simulink model "MIL_VehicleTestEnvironment_MG_DCT_1"  (Simulink 10.0)
settings: Solver=ode4  StartTime=0.0  StopTime=20  FixedStep=0.001  MaxStep=0.005  RelTol=1e-3  EnableMultiTasking=on
undefined symbols (not defined in the file or in its folder): Clu1FricCoefMap, Clu2FricCoefMap, CluSoln1LineI, CluSoln1LineP, CluSoln2LineI, CluSoln2LineP, DiffDampCoef, EngFuelCnsPerSecMapCns, EngFuelCnsPerSecMapSpdIndx, EngFuelCnsPerSecMapThrtIndx, EngIdleSpd, EngSpdMax, EngTqExtChartc, EngTqMapSpdIndx, EngTqMapThrtIndx, EngTqMapTq, EngTqMax, Fork13ActrAr, Fork1PosnA, Fork1PosnB, Fork1PosnNeut, Fork1PosnSyncA, Fork1PosnSyncB, Fork24ActrAr, Fork2PosnA, Fork2PosnB, Fork2PosnNeut, Fork2PosnSyncA, Fork2PosnSyncB, Fork3PosnA, Fork3PosnB, Fork3PosnNeut, Fork3PosnSyncA, Fork3PosnSyncB, Fork4PosnA, Fork4PosnB, Fork4PosnNeut, Fork4PosnSyncA, Fork4PosnSyncB, Fork6RActrAr, ForkN5ActrAr, GearRat, HalfShafInrt, IdleGearInrt, InpShaf1DampCoef, InpShaf2DampCoef, OutpShaf1DampCoef, OutpShaf2DampCoef, ShiftSoln1LineI, ShiftSoln1LineP, ShiftSoln2LineI, ShiftSoln2LineP, SynrDiaBig, SynrDplDog, SynrDplEngd, SynrDplFinshd, SynrDplSync, SynrFricCoef, VBS1R, VBS2R ... (+6)
libraries: fl_lib x71, nesl_utility x34, sdl_lib x20, fl_ps_legacy_lib x8, simulink x5
(part 2 of 2)

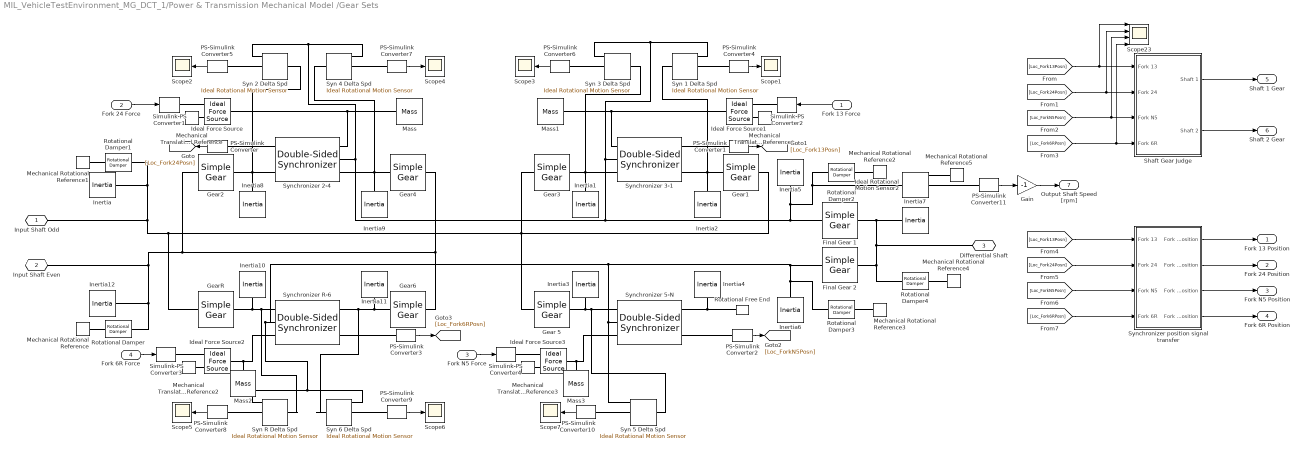
== system MIL_VehicleTestEnvironment_MG_DCT_1/Power & Transmission Mechanical Model /Gear Sets ==
  Fork 13 Force : Inport
  Fork 24 Force : Inport  Port=2
  Fork N5 Force : Inport  Port=3
  Fork 6R Force : Inport  Port=4
  Final Gear 1 : sdl_lib/Gears/Simple Gear  ratio=FinlGearRat1  rotation_direction=2  friction_model=1  T_noload=0.1 N*m  T_nom=5 N*m  efficiency_nom=0.8  efficiency=0.8  mu_visc=[ 0 0 ] N*m/(rad/s)  w_thr=0.01 rad/s  pwr_thr=0.001 W  enable_faults=simscape.enum.onoff.off  efficiency_fault=0.05  external_fault=simscape.enum.onoff.off  temporal_fault=simscape.enum.onoff.off  fault_time=5 s  fault_angles=pi / 12 rad  report_fault=1  temperature_TLU=[280, 300, 320] K  load_TLU=[1, 5, 10] N*m  efficiency_TLU=[.95, .9, .85]  efficiency_TLU2=[.85, .8, .75; .95, .9, .85; .85, .8, .7]  thermal_mass=50 J/K  T_init=300 K
  Final Gear 2 : sdl_lib/Gears/Simple Gear  ratio=FinlGearRat2  rotation_direction=2  friction_model=1  T_noload=0.1 N*m  T_nom=5 N*m  efficiency_nom=0.8  efficiency=0.8  mu_visc=[ 0 0 ] N*m/(rad/s)  w_thr=0.01 rad/s  pwr_thr=0.001 W  enable_faults=simscape.enum.onoff.off  efficiency_fault=0.05  external_fault=simscape.enum.onoff.off  temporal_fault=simscape.enum.onoff.off  fault_time=5 s  fault_angles=pi / 12 rad  report_fault=1  temperature_TLU=[280, 300, 320] K  load_TLU=[1, 5, 10] N*m  efficiency_TLU=[.95, .9, .85]  efficiency_TLU2=[.85, .8, .75; .95, .9, .85; .85, .8, .7]  thermal_mass=50 J/K  T_init=300 K
  Gain : Gain  Gain=-1
  Gear 5 : sdl_lib/Gears/Simple Gear  ratio=GearRat(5)  rotation_direction=2  friction_model=1  T_noload=0.1 N*m  T_nom=5 N*m  efficiency_nom=0.8  efficiency=0.8  mu_visc=[ 0 0 ] N*m/(rad/s)  w_thr=0.01 rad/s  pwr_thr=0.001 W  enable_faults=simscape.enum.onoff.off  efficiency_fault=0.05  external_fault=simscape.enum.onoff.off  temporal_fault=simscape.enum.onoff.off  fault_time=5 s  fault_angles=pi / 12 rad  report_fault=1  temperature_TLU=[280, 300, 320] K  load_TLU=[1, 5, 10] N*m  efficiency_TLU=[.95, .9, .85]  efficiency_TLU2=[.85, .8, .75; .95, .9, .85; .85, .8, .7]  thermal_mass=50 J/K  T_init=300 K
  Gear1 : sdl_lib/Gears/Simple Gear  ratio=GearRat(1)  rotation_direction=2  friction_model=1  T_noload=0.1 N*m  T_nom=5 N*m  efficiency_nom=0.8  efficiency=0.8  mu_visc=[ 0 0 ] N*m/(rad/s)  w_thr=0.01 rad/s  pwr_thr=0.001 W  enable_faults=simscape.enum.onoff.off  efficiency_fault=0.05  external_fault=simscape.enum.onoff.off  temporal_fault=simscape.enum.onoff.off  fault_time=5 s  fault_angles=pi / 12 rad  report_fault=1  temperature_TLU=[280, 300, 320] K  load_TLU=[1, 5, 10] N*m  efficiency_TLU=[.95, .9, .85]  efficiency_TLU2=[.85, .8, .75; .95, .9, .85; .85, .8, .7]  thermal_mass=50 J/K  T_init=300 K
  Gear2 : sdl_lib/Gears/Simple Gear  ratio=GearRat(2)  rotation_direction=2  friction_model=1  T_noload=0.1 N*m  T_nom=5 N*m  efficiency_nom=0.8  efficiency=0.8  mu_visc=[ 0 0 ] N*m/(rad/s)  w_thr=0.01 rad/s  pwr_thr=0.001 W  enable_faults=simscape.enum.onoff.off  efficiency_fault=0.05  external_fault=simscape.enum.onoff.off  temporal_fault=simscape.enum.onoff.off  fault_time=5 s  fault_angles=pi / 12 rad  report_fault=1  temperature_TLU=[280, 300, 320] K  load_TLU=[1, 5, 10] N*m  efficiency_TLU=[.95, .9, .85]  efficiency_TLU2=[.85, .8, .75; .95, .9, .85; .85, .8, .7]  thermal_mass=50 J/K  T_init=300 K
  Gear3 : sdl_lib/Gears/Simple Gear  ratio=GearRat(3)  rotation_direction=2  friction_model=1  T_noload=0.1 N*m  T_nom=5 N*m  efficiency_nom=0.8  efficiency=0.8  mu_visc=[ 0 0 ] N*m/(rad/s)  w_thr=0.01 rad/s  pwr_thr=0.001 W  enable_faults=simscape.enum.onoff.off  efficiency_fault=0.05  external_fault=simscape.enum.onoff.off  temporal_fault=simscape.enum.onoff.off  fault_time=5 s  fault_angles=pi / 12 rad  report_fault=1  temperature_TLU=[280, 300, 320] K  load_TLU=[1, 5, 10] N*m  efficiency_TLU=[.95, .9, .85]  efficiency_TLU2=[.85, .8, .75; .95, .9, .85; .85, .8, .7]  thermal_mass=50 J/K  T_init=300 K
  Gear4 : sdl_lib/Gears/Simple Gear  ratio=GearRat(4)  rotation_direction=2  friction_model=1  T_noload=0.1 N*m  T_nom=5 N*m  efficiency_nom=0.8  efficiency=0.8  mu_visc=[ 0 0 ] N*m/(rad/s)  w_thr=0.01 rad/s  pwr_thr=0.001 W  enable_faults=simscape.enum.onoff.off  efficiency_fault=0.05  external_fault=simscape.enum.onoff.off  temporal_fault=simscape.enum.onoff.off  fault_time=5 s  fault_angles=pi / 12 rad  report_fault=1  temperature_TLU=[280, 300, 320] K  load_TLU=[1, 5, 10] N*m  efficiency_TLU=[.95, .9, .85]  efficiency_TLU2=[.85, .8, .75; .95, .9, .85; .85, .8, .7]  thermal_mass=50 J/K  T_init=300 K
  Gear6 : sdl_lib/Gears/Simple Gear  ratio=GearRat(6)  rotation_direction=2  friction_model=1  T_noload=0.1 N*m  T_nom=5 N*m  efficiency_nom=0.8  efficiency=0.8  mu_visc=[ 0 0 ] N*m/(rad/s)  w_thr=0.01 rad/s  pwr_thr=0.001 W  enable_faults=simscape.enum.onoff.off  efficiency_fault=0.05  external_fault=simscape.enum.onoff.off  temporal_fault=simscape.enum.onoff.off  fault_time=5 s  fault_angles=pi / 12 rad  report_fault=1  temperature_TLU=[280, 300, 320] K  load_TLU=[1, 5, 10] N*m  efficiency_TLU=[.95, .9, .85]  efficiency_TLU2=[.85, .8, .75; .95, .9, .85; .85, .8, .7]  thermal_mass=50 J/K  T_init=300 K
  GearR : sdl_lib/Gears/Simple Gear  ratio=GearRat(7)  rotation_direction=1  friction_model=1  T_noload=0.1 N*m  T_nom=5 N*m  efficiency_nom=0.8  efficiency=0.8  mu_visc=[ 0 0 ] N*m/(rad/s)  w_thr=0.01 rad/s  pwr_thr=0.001 W  enable_faults=simscape.enum.onoff.off  efficiency_fault=0.05  external_fault=simscape.enum.onoff.off  temporal_fault=simscape.enum.onoff.off  fault_time=5 s  fault_angles=pi / 12 rad  report_fault=1  temperature_TLU=[280, 300, 320] K  load_TLU=[1, 5, 10] N*m  efficiency_TLU=[.95, .9, .85]  efficiency_TLU2=[.85, .8, .75; .95, .9, .85; .85, .8, .7]  thermal_mass=50 J/K  T_init=300 K
  Ideal Force Source{,1..3} (4 alike) : fl_lib/Mechanical/Mechanical Sources/Ideal Force Source
  Ideal Rotational Motion Sensor2 : fl_lib/Mechanical/Mechanical Sensors/Ideal Rotational Motion Sensor  wrap_angle=simscape.enum.onoff.off  offset=0 rad
  Inertia : fl_lib/Mechanical/Rotational Elements/Inertia  inertia=InpShaf1Inrt kg*m^2  w_specify=off  w_priority=High  w=0 rad/s  w_nominal_specify=off  w_nominal_unit=rad/s  w_nominal_value=1  t_specify=off  t_priority=High  t=0 N*m  t_nominal_specify=off  t_nominal_unit=N*m  t_nominal_value=1
  Inertia1 : fl_lib/Mechanical/Rotational Elements/Inertia  inertia=IdleGearInrt(3) kg*m^2  w_specify=off  w_priority=High  w=0 rad/s  w_nominal_specify=off  w_nominal_unit=rad/s  w_nominal_value=1  t_specify=off  t_priority=High  t=0 N*m  t_nominal_specify=off  t_nominal_unit=N*m  t_nominal_value=1
  Inertia10 : fl_lib/Mechanical/Rotational Elements/Inertia  inertia=IdleGearInrt(7) kg*m^2  w_specify=off  w_priority=High  w=0 rad/s  w_nominal_specify=off  w_nominal_unit=rad/s  w_nominal_value=1  t_specify=off  t_priority=High  t=0 N*m  t_nominal_specify=off  t_nominal_unit=N*m  t_nominal_value=1
  Inertia11 : fl_lib/Mechanical/Rotational Elements/Inertia  inertia=IdleGearInrt(6) kg*m^2  w_specify=off  w_priority=High  w=0 rad/s  w_nominal_specify=off  w_nominal_unit=rad/s  w_nominal_value=1  t_specify=off  t_priority=High  t=0 N*m  t_nominal_specify=off  t_nominal_unit=N*m  t_nominal_value=1
  Inertia12 : fl_lib/Mechanical/Rotational Elements/Inertia  inertia=InpShaf2Inrt kg*m^2  w_specify=off  w_priority=High  w=0 rad/s  w_nominal_specify=off  w_nominal_unit=rad/s  w_nominal_value=1  t_specify=off  t_priority=High  t=0 N*m  t_nominal_specify=off  t_nominal_unit=N*m  t_nominal_value=1
  Inertia2 : fl_lib/Mechanical/Rotational Elements/Inertia  inertia=IdleGearInrt(1) kg*m^2  w_specify=off  w_priority=High  w=0 rad/s  w_nominal_specify=off  w_nominal_unit=rad/s  w_nominal_value=1  t_specify=off  t_priority=High  t=0 N*m  t_nominal_specify=off  t_nominal_unit=N*m  t_nominal_value=1
  Inertia3 : fl_lib/Mechanical/Rotational Elements/Inertia  inertia=IdleGearInrt(5) kg*m^2  w_specify=off  w_priority=High  w=0 rad/s  w_nominal_specify=off  w_nominal_unit=rad/s  w_nominal_value=1  t_specify=off  t_priority=High  t=0 N*m  t_nominal_specify=off  t_nominal_unit=N*m  t_nominal_value=1
  Inertia4 : fl_lib/Mechanical/Rotational Elements/Inertia  inertia=0.001 kg*m^2  w_specify=off  w_priority=High  w=0 rad/s  w_nominal_specify=off  w_nominal_unit=rad/s  w_nominal_value=1  t_specify=off  t_priority=High  t=0 N*m  t_nominal_specify=off  t_nominal_unit=N*m  t_nominal_value=1
  Inertia5 : fl_lib/Mechanical/Rotational Elements/Inertia  inertia=OutpShaf1Inrt kg*m^2  w_specify=off  w_priority=High  w=0 rad/s  w_nominal_specify=off  w_nominal_unit=rad/s  w_nominal_value=1  t_specify=off  t_priority=High  t=0 N*m  t_nominal_specify=off  t_nominal_unit=N*m  t_nominal_value=1
  Inertia6 : fl_lib/Mechanical/Rotational Elements/Inertia  inertia=OutpShaf2Inrt kg*m^2  w_specify=off  w_priority=High  w=0 rad/s  w_nominal_specify=off  w_nominal_unit=rad/s  w_nominal_value=1  t_specify=off  t_priority=High  t=0 N*m  t_nominal_specify=off  t_nominal_unit=N*m  t_nominal_value=1
  Inertia7 : fl_lib/Mechanical/Rotational Elements/Inertia  inertia=DiffInrt kg*m^2  w_specify=off  w_priority=High  w=0 rad/s  w_nominal_specify=off  w_nominal_unit=rad/s  w_nominal_value=1  t_specify=off  t_priority=High  t=0 N*m  t_nominal_specify=off  t_nominal_unit=N*m  t_nominal_value=1
  Inertia8 : fl_lib/Mechanical/Rotational Elements/Inertia  inertia=IdleGearInrt(2) kg*m^2  w_specify=off  w_priority=High  w=0 rad/s  w_nominal_specify=off  w_nominal_unit=rad/s  w_nominal_value=1  t_specify=off  t_priority=High  t=0 N*m  t_nominal_specify=off  t_nominal_unit=N*m  t_nominal_value=1
  Inertia9 : fl_lib/Mechanical/Rotational Elements/Inertia  inertia=IdleGearInrt(4) kg*m^2  w_specify=off  w_priority=High  w=0 rad/s  w_nominal_specify=off  w_nominal_unit=rad/s  w_nominal_value=1  t_specify=off  t_priority=High  t=0 N*m  t_nominal_specify=off  t_nominal_unit=N*m  t_nominal_value=1
  Mass{,1..3} (4 alike) : fl_lib/Mechanical/Translational Elements/Mass  mass=1 kg  v_specify=off  v_priority=High  v=0 m/s  v_nominal_specify=off  v_nominal_unit=m/s  v_nominal_value=1  f_specify=off  f_priority=High  f=0 N  f_nominal_specify=off  f_nominal_unit=N  f_nominal_value=1
  Mechanical Rotational Reference{,1..5} (6 alike) : fl_lib/Mechanical/Rotational Elements/Mechanical Rotational Reference
  Mechanical Translational Reference{,1..3} (4 alike) : fl_lib/Mechanical/Translational Elements/Mechanical Translational Reference
  PS-Simulink Converter{,1..3} (4 alike) : nesl_utility/PS-Simulink Converter  PhysicalDomain=network_engine_domain  SubClassName=ps_output  LeftPortType=input  RightPortType=output  PseudoPeriodic=off  Frequencies=[]  Unit=mm  AffineConversion=off
  PS-Simulink Converter{4..11} (8 alike) : nesl_utility/PS-Simulink Converter  PhysicalDomain=network_engine_domain  SubClassName=ps_output  LeftPortType=input  RightPortType=output  PseudoPeriodic=off  Frequencies=[]  Unit=rpm  AffineConversion=off
  Rotational Damper : fl_lib/Mechanical/Rotational Elements/Rotational Damper  D=InpShaf2DampCoef N*m/(rad/s)  w_specify=off  w_priority=High  w=0 rad/s  w_nominal_specify=off  w_nominal_unit=rad/s  w_nominal_value=1  t_specify=off  t_priority=High  t=0 N*m  t_nominal_specify=off  t_nominal_unit=N*m  t_nominal_value=1
  Rotational Damper1 : fl_lib/Mechanical/Rotational Elements/Rotational Damper  D=InpShaf1DampCoef N*m/(rad/s)  w_specify=off  w_priority=High  w=0 rad/s  w_nominal_specify=off  w_nominal_unit=rad/s  w_nominal_value=1  t_specify=off  t_priority=High  t=0 N*m  t_nominal_specify=off  t_nominal_unit=N*m  t_nominal_value=1
  Rotational Damper2 : fl_lib/Mechanical/Rotational Elements/Rotational Damper  D=OutpShaf1DampCoef N*m/(rad/s)  w_specify=off  w_priority=High  w=0 rad/s  w_nominal_specify=off  w_nominal_unit=rad/s  w_nominal_value=1  t_specify=off  t_priority=High  t=0 N*m  t_nominal_specify=off  t_nominal_unit=N*m  t_nominal_value=1
  Rotational Damper3 : fl_lib/Mechanical/Rotational Elements/Rotational Damper  D=OutpShaf2DampCoef N*m/(rad/s)  w_specify=off  w_priority=High  w=0 rad/s  w_nominal_specify=off  w_nominal_unit=rad/s  w_nominal_value=1  t_specify=off  t_priority=High  t=0 N*m  t_nominal_specify=off  t_nominal_unit=N*m  t_nominal_value=1
  Rotational Damper4 : fl_lib/Mechanical/Rotational Elements/Rotational Damper  D=DiffDampCoef N*m/(rad/s)  w_specify=off  w_priority=High  w=0 rad/s  w_nominal_specify=off  w_nominal_unit=rad/s  w_nominal_value=1  t_specify=off  t_priority=High  t=0 N*m  t_nominal_specify=off  t_nominal_unit=N*m  t_nominal_value=1
  Rotational Free End : fl_lib/Mechanical/Rotational Elements/Rotational Free End  w_specify=off  w_priority=None  w=0 rad/s  w_nominal_specify=off  w_nominal_unit=rad/s  w_nominal_value=1
      settings: SourceProductBaseCode=SS
  Scope{1..7} (7 alike) : Scope
  Scope23 : Scope  NumInputPorts=4
  "Shaft Gear Judge " : Subsystem
  Simulink-PS Converter{1..4} (4 alike) : nesl_utility/Simulink-PS Converter  PhysicalDomain=network_engine_domain  SubClassName=ps_input  LeftPortType=input  RightPortType=output  PseudoPeriodic=off  Frequencies=[]  NoiseDistribution=none  NoiseParameters=[]  Unit=N  AffineConversion=off  FilteringAndDerivatives=zero  SimscapeFilterOrder=1  InputFilterTimeConstant=0.001  UdotUserProvided=1
  Syn 1 Delta Spd : fl_lib/Mechanical/Mechanical Sensors/Ideal Rotational Motion Sensor  wrap_angle=simscape.enum.onoff.off  offset=0 rad
  Syn 2 Delta Spd : fl_lib/Mechanical/Mechanical Sensors/Ideal Rotational Motion Sensor  wrap_angle=simscape.enum.onoff.off  offset=0 rad
  Syn 3 Delta Spd : fl_lib/Mechanical/Mechanical Sensors/Ideal Rotational Motion Sensor  wrap_angle=simscape.enum.onoff.off  offset=0 rad
  Syn 4 Delta Spd : fl_lib/Mechanical/Mechanical Sensors/Ideal Rotational Motion Sensor  wrap_angle=simscape.enum.onoff.off  offset=0 rad
  Syn 5 Delta Spd : fl_lib/Mechanical/Mechanical Sensors/Ideal Rotational Motion Sensor  wrap_angle=simscape.enum.onoff.off  offset=0 rad
  Syn 6 Delta Spd : fl_lib/Mechanical/Mechanical Sensors/Ideal Rotational Motion Sensor  wrap_angle=simscape.enum.onoff.off  offset=0 rad
  Syn R Delta Spd : fl_lib/Mechanical/Mechanical Sensors/Ideal Rotational Motion Sensor  wrap_angle=simscape.enum.onoff.off  offset=0 rad
  Synchronizer 2-4 : sdl_lib/Clutches/Double-Sided Synchronizer  d_o=SynrDiaBig*2 m  d_i=SynrDiaSmal m  theta=SynrConeAngl deg  friction_model=2  mu_w_vector=SynrFricCoef(:,1) rad/s  mu_temperature_TLU=[280, 300, 320] K  mu_static=SynrFricCoef(1,2)+0.05  mu_static_vector=[.4, .38, .36]  mu_coulomb=0.3  mu_coulomb_vector=SynrFricCoef(:,2)  mu_coulomb_temp_vector=[.3, .28, .25]  mu_coulomb_matrix=[.34, .32, .3; .3, .28, .25; .25, .2, .15]  mu_interp_method=1  mu_extrap_method=1  w_tol=0.001 rad/s  force_min=1 N  model=1  max_torque=1000 N*m  torque_temperature_TLU=[280, 300, 320] K  max_torque_vector=[1000, 1050, 1000] N*m  torque_interp_method=1  torque_extrap_method=1  radius=200 mm  n_teeth=6  clutch_backlash=10 deg  clutch_stiffness=1e+7 N*m/rad  clutch_damping=100 N*m/(rad/s)  fric_coeff=0.05  peak_force=SynrDetnForMax N  width=SynrNotchWidth mm  detent_visc_fric_transl=0.1 N/(m/s)  friction_ratio=0.01  v_thr=0.05 m/s  engagement_speed=1 rpm  dog_clutch_ring_hub_gap=SynrDplDog mm  engagement_overlap=SynrDplEngd-SynrDplDog mm  tooth_height=SynrDplFinshd-SynrDplDog mm  cone_clutch_ring_hub_gap=SynrDplSync mm  dog_clutch_transl_stiffness=1e+6 N/m  cone_clutch_transl_stiffness=1e+6 N/m  dog_clutch_transl_damping=1000 N/(m/s)  cone_clutch_transl_damping=1000 N/(m/s)  dog_clutch_visc_fric_transl=SynrVcosFricCoeff N/(m/s)  initial_state_locked=3  dog_clutch_init_pos=0 mm  cone_clutch_init_pos=0 mm  init_rel_angle_A=0 deg  init_rel_angle_B=0 deg  thermal_mass=100 kJ/K  T_init=300 K
      settings: SourceProductBaseCode=LD  InternalSimscapePortConfiguration="{\"Bottom\":[],\"Left\":[{\"id\":\"S\",\"label\":\"S\",\"type\":\"foundation.mechanical.translational.translational\"},{\"id\":\"R\",\"label\":\"R\",\"type\":\"foundation.mechanical.rotational.rotational\"},{\"id\":\"HA\",\"label\":\"HA\",\"type\":\"foundation.mechanical.rotational.rotational\"}],\"Right\":[{\"id\":\"X1\",\"label\":\"X1\",\"type\":\"output\"},{\"id\":\"X2\",\"label\":\"X2\",\"type\":\"output\"},{\"id\":\"HB\",\"label\":\"HB\",\"type\":\"foundation.mechanical.rotational.rotational\"}],\"Top\":[]}"
  Synchronizer 3-1 : sdl_lib/Clutches/Double-Sided Synchronizer  d_o=SynrDiaBig m  d_i=SynrDiaSmal m  theta=SynrConeAngl deg  friction_model=2  mu_w_vector=SynrFricCoef(:,1) rad/s  mu_temperature_TLU=[280, 300, 320] K  mu_static=SynrFricCoef(1,2)+0.05  mu_static_vector=[.4, .38, .36]  mu_coulomb=0.3  mu_coulomb_vector=SynrFricCoef(:,2)  mu_coulomb_temp_vector=[.3, .28, .25]  mu_coulomb_matrix=[.34, .32, .3; .3, .28, .25; .25, .2, .15]  mu_interp_method=1  mu_extrap_method=1  w_tol=0.001 rad/s  force_min=1 N  model=1  max_torque=1000 N*m  torque_temperature_TLU=[280, 300, 320] K  max_torque_vector=[1000, 1050, 1000] N*m  torque_interp_method=1  torque_extrap_method=1  radius=200 mm  n_teeth=6  clutch_backlash=10 deg  clutch_stiffness=1e+7 N*m/rad  clutch_damping=100 N*m/(rad/s)  fric_coeff=0.05  peak_force=SynrDetnForMax N  width=SynrNotchWidth mm  detent_visc_fric_transl=0.1 N/(m/s)  friction_ratio=0.01  v_thr=0.05 m/s  engagement_speed=1 rpm  dog_clutch_ring_hub_gap=SynrDplDog mm  engagement_overlap=SynrDplEngd-SynrDplDog mm  tooth_height=SynrDplFinshd-SynrDplDog mm  cone_clutch_ring_hub_gap=SynrDplSync mm  dog_clutch_transl_stiffness=1e+6 N/m  cone_clutch_transl_stiffness=1e+6 N/m  dog_clutch_transl_damping=1000 N/(m/s)  cone_clutch_transl_damping=1000 N/(m/s)  dog_clutch_visc_fric_transl=SynrVcosFricCoeff N/(m/s)  initial_state_locked=3  dog_clutch_init_pos=0 mm  cone_clutch_init_pos=0 mm  init_rel_angle_A=0 deg  init_rel_angle_B=0 deg  thermal_mass=100 kJ/K  T_init=300 K
      settings: SourceProductBaseCode=LD  InternalSimscapePortConfiguration="{\"Bottom\":[],\"Left\":[{\"id\":\"S\",\"label\":\"S\",\"type\":\"foundation.mechanical.translational.translational\"},{\"id\":\"R\",\"label\":\"R\",\"type\":\"foundation.mechanical.rotational.rotational\"},{\"id\":\"HA\",\"label\":\"HA\",\"type\":\"foundation.mechanical.rotational.rotational\"}],\"Right\":[{\"id\":\"X1\",\"label\":\"X1\",\"type\":\"output\"},{\"id\":\"X2\",\"label\":\"X2\",\"type\":\"output\"},{\"id\":\"HB\",\"label\":\"HB\",\"type\":\"foundation.mechanical.rotational.rotational\"}],\"Top\":[]}"
  Synchronizer 5-N : sdl_lib/Clutches/Double-Sided Synchronizer  d_o=SynrDiaBig m  d_i=SynrDiaSmal m  theta=SynrConeAngl deg  friction_model=2  mu_w_vector=SynrFricCoef(:,1) rad/s  mu_temperature_TLU=[280, 300, 320] K  mu_static=SynrFricCoef(1,2)+0.05  mu_static_vector=[.4, .38, .36]  mu_coulomb=0.3  mu_coulomb_vector=SynrFricCoef(:,2)  mu_coulomb_temp_vector=[.3, .28, .25]  mu_coulomb_matrix=[.34, .32, .3; .3, .28, .25; .25, .2, .15]  mu_interp_method=1  mu_extrap_method=1  w_tol=0.001 rad/s  force_min=1 N  model=1  max_torque=1000 N*m  torque_temperature_TLU=[280, 300, 320] K  max_torque_vector=[1000, 1050, 1000] N*m  torque_interp_method=1  torque_extrap_method=1  radius=200 mm  n_teeth=6  clutch_backlash=10 deg  clutch_stiffness=1e+7 N*m/rad  clutch_damping=100 N*m/(rad/s)  fric_coeff=0.05  peak_force=SynrDetnForMax N  width=SynrNotchWidth mm  detent_visc_fric_transl=0.1 N/(m/s)  friction_ratio=0.01  v_thr=0.05 m/s  engagement_speed=1 rpm  dog_clutch_ring_hub_gap=SynrDplDog mm  engagement_overlap=SynrDplEngd-SynrDplDog mm  tooth_height=SynrDplFinshd-SynrDplDog mm  cone_clutch_ring_hub_gap=SynrDplSync mm  dog_clutch_transl_stiffness=1e+6 N/m  cone_clutch_transl_stiffness=1e+6 N/m  dog_clutch_transl_damping=1000 N/(m/s)  cone_clutch_transl_damping=1000 N/(m/s)  dog_clutch_visc_fric_transl=SynrVcosFricCoeff N/(m/s)  initial_state_locked=3  dog_clutch_init_pos=0 mm  cone_clutch_init_pos=0 mm  init_rel_angle_A=0 deg  init_rel_angle_B=0 deg  thermal_mass=100 kJ/K  T_init=300 K
      settings: SourceProductBaseCode=LD  InternalSimscapePortConfiguration="{\"Bottom\":[],\"Left\":[{\"id\":\"S\",\"label\":\"S\",\"type\":\"foundation.mechanical.translational.translational\"},{\"id\":\"R\",\"label\":\"R\",\"type\":\"foundation.mechanical.rotational.rotational\"},{\"id\":\"HA\",\"label\":\"HA\",\"type\":\"foundation.mechanical.rotational.rotational\"}],\"Right\":[{\"id\":\"X1\",\"label\":\"X1\",\"type\":\"output\"},{\"id\":\"X2\",\"label\":\"X2\",\"type\":\"output\"},{\"id\":\"HB\",\"label\":\"HB\",\"type\":\"foundation.mechanical.rotational.rotational\"}],\"Top\":[]}"
  Synchronizer R-6 : sdl_lib/Clutches/Double-Sided Synchronizer  d_o=SynrDiaBig m  d_i=SynrDiaSmal m  theta=SynrConeAngl deg  friction_model=2  mu_w_vector=SynrFricCoef(:,1) rad/s  mu_temperature_TLU=[280, 300, 320] K  mu_static=SynrFricCoef(1,2)+0.05  mu_static_vector=[.4, .38, .36]  mu_coulomb=0.3  mu_coulomb_vector=SynrFricCoef(:,2)  mu_coulomb_temp_vector=[.3, .28, .25]  mu_coulomb_matrix=[.34, .32, .3; .3, .28, .25; .25, .2, .15]  mu_interp_method=1  mu_extrap_method=1  w_tol=0.001 rad/s  force_min=1 N  model=1  max_torque=1000 N*m  torque_temperature_TLU=[280, 300, 320] K  max_torque_vector=[1000, 1050, 1000] N*m  torque_interp_method=1  torque_extrap_method=1  radius=200 mm  n_teeth=6  clutch_backlash=10 deg  clutch_stiffness=1e+7 N*m/rad  clutch_damping=100 N*m/(rad/s)  fric_coeff=0.05  peak_force=SynrDetnForMax N  width=SynrNotchWidth mm  detent_visc_fric_transl=0.1 N/(m/s)  friction_ratio=0.01  v_thr=0.05 m/s  engagement_speed=1 rpm  dog_clutch_ring_hub_gap=SynrDplDog mm  engagement_overlap=SynrDplEngd-SynrDplDog mm  tooth_height=SynrDplFinshd-SynrDplDog mm  cone_clutch_ring_hub_gap=SynrDplSync mm  dog_clutch_transl_stiffness=1e+6 N/m  cone_clutch_transl_stiffness=1e+6 N/m  dog_clutch_transl_damping=1000 N/(m/s)  cone_clutch_transl_damping=1000 N/(m/s)  dog_clutch_visc_fric_transl=SynrVcosFricCoeff N/(m/s)  initial_state_locked=3  dog_clutch_init_pos=0 mm  cone_clutch_init_pos=0 mm  init_rel_angle_A=0 deg  init_rel_angle_B=0 deg  thermal_mass=100 kJ/K  T_init=300 K
      settings: SourceProductBaseCode=LD  InternalSimscapePortConfiguration="{\"Bottom\":[],\"Left\":[{\"id\":\"S\",\"label\":\"S\",\"type\":\"foundation.mechanical.translational.translational\"},{\"id\":\"R\",\"label\":\"R\",\"type\":\"foundation.mechanical.rotational.rotational\"},{\"id\":\"HA\",\"label\":\"HA\",\"type\":\"foundation.mechanical.rotational.rotational\"}],\"Right\":[{\"id\":\"X1\",\"label\":\"X1\",\"type\":\"output\"},{\"id\":\"X2\",\"label\":\"X2\",\"type\":\"output\"},{\"id\":\"HB\",\"label\":\"HB\",\"type\":\"foundation.mechanical.rotational.rotational\"}],\"Top\":[]}"
  Synchronizer position signal transfer : Subsystem
  Input Shaft Odd : PMIOPort  Side=Left
  Input Shaft Even : PMIOPort  Port=2  Side=Left
  Differential Shaft : PMIOPort  Port=3  Side=Right
  Fork 13 Position : Outport  VectorParamsAs1DForOutWhenUnconnected=off
  Fork 24 Position : Outport  Port=2  VectorParamsAs1DForOutWhenUnconnected=off
  Fork N5 Position : Outport  Port=3  VectorParamsAs1DForOutWhenUnconnected=off
  Fork 6R Position : Outport  Port=4  VectorParamsAs1DForOutWhenUnconnected=off
  Shaft 1 Gear : Outport  Port=5  VectorParamsAs1DForOutWhenUnconnected=off
  Shaft 2 Gear : Outport  Port=6  VectorParamsAs1DForOutWhenUnconnected=off
  Output Shaft Speed [rpm] : Outport  Port=7  VectorParamsAs1DForOutWhenUnconnected=off
  wires:
  PS-Simulink Converter/1 -> [Loc_Fork24Posn]
  PS-Simulink Converter1/1 -> [Loc_Fork13Posn]
  PS-Simulink Converter2/1 -> [Loc_ForkN5Posn]
  [Loc_Fork13Posn] -> Scope23/1, "Shaft Gear Judge "/1(Fork 13)
  [Loc_Fork24Posn] -> Scope23/2, "Shaft Gear Judge "/2(Fork 24)
  [Loc_ForkN5Posn] -> Scope23/3, "Shaft Gear Judge "/3(Fork N5)
  [Loc_Fork6RPosn] -> Scope23/4, "Shaft Gear Judge "/4(Fork 6R)
  "Shaft Gear Judge "/1(Shaft 1) -> Shaft 1 Gear/1
  "Shaft Gear Judge "/2(Shaft 2) -> Shaft 2 Gear/1
  PS-Simulink Converter3/1 -> [Loc_Fork6RPosn]
  Fork 6R Force/1 -> Simulink-PS Converter3/1
  Fork N5 Force/1 -> Simulink-PS Converter4/1
  [Loc_Fork24Posn] -> Synchronizer position signal transfer/2(Fork 24)
  [Loc_ForkN5Posn] -> Synchronizer position signal transfer/3(Fork N5)
  [Loc_Fork6RPosn] -> Synchronizer position signal transfer/4(Fork 6R)
  [Loc_Fork13Posn] -> Synchronizer position signal transfer/1(Fork 13)
  Synchronizer position signal transfer/1(Fork 13 Position) -> Fork 13 Position/1
  Synchronizer position signal transfer/3(Fork N5 Position) -> Fork N5 Position/1
  Synchronizer position signal transfer/2(Fork 24 Position) -> Fork 24 Position/1
  Synchronizer position signal transfer/4(Fork 6R Position) -> Fork 6R Position/1
  PS-Simulink Converter4/1 -> Scope1/1
  PS-Simulink Converter6/1 -> Scope3/1
  PS-Simulink Converter5/1 -> Scope2/1
  PS-Simulink Converter7/1 -> Scope4/1
  PS-Simulink Converter8/1 -> Scope5/1
  PS-Simulink Converter9/1 -> Scope6/1
  PS-Simulink Converter10/1 -> Scope7/1
  Fork 24 Force/1 -> Simulink-PS Converter1/1
  Fork 13 Force/1 -> Simulink-PS Converter2/1
  PS-Simulink Converter11/1 -> Gain/1
  Gain/1 -> Output Shaft Speed [rpm]/1
  connections:
  Gear 5/LConn1 -- Gear1/LConn1 -- Gear3/LConn1 -- GearR/LConn1 -- Rotational Damper1/LConn1 -- Inertia/LConn1 -- Input Shaft Odd/RConn1
  Gear3/RConn1 -- Syn 3 Delta Spd/LConn1 -- Inertia1/LConn1 -- Synchronizer 3-1/LConn3
  Gear1/RConn1 -- Syn 1 Delta Spd/LConn1 -- Synchronizer 3-1/RConn3 -- Inertia2/LConn1
  Gear 5/RConn1 -- Syn 5 Delta Spd/LConn1 -- Synchronizer 5-N/LConn3 -- Inertia3/LConn1
  Final Gear 1/LConn1 -- Syn 2 Delta Spd/RConn1 -- Syn 4 Delta Spd/RConn1 -- Synchronizer 2-4/LConn2 -- Syn 3 Delta Spd/RConn1 -- Syn 1 Delta Spd/RConn1 -- Synchronizer 3-1/LConn2 -- Ideal Rotational Motion Sensor2/LConn1 -- Rotational Damper2/LConn1 -- Inertia5/LConn1
  Syn 6 Delta Spd/RConn1 -- Syn R Delta Spd/RConn1 -- Synchronizer R-6/LConn2 -- Syn 5 Delta Spd/RConn1 -- Synchronizer 5-N/LConn2 -- Rotational Damper3/LConn1 -- Inertia6/LConn1 -- Final Gear 2/LConn1
  Differential Shaft/RConn1 -- Final Gear 1/RConn1 -- Inertia7/LConn1 -- Rotational Damper4/LConn1 -- Final Gear 2/RConn1
  Gear4/RConn1 -- Syn 4 Delta Spd/LConn1 -- Synchronizer 2-4/LConn3 -- Inertia9/LConn1
  Synchronizer 2-4/RConn3 -- Syn 2 Delta Spd/LConn1 -- Inertia8/LConn1 -- Gear2/RConn1
  GearR/RConn1 -- Syn R Delta Spd/LConn1 -- Synchronizer R-6/LConn3 -- Inertia10/LConn1
  Syn 6 Delta Spd/LConn1 -- Synchronizer R-6/RConn3 -- Gear6/RConn1 -- Inertia11/LConn1
  Gear4/LConn1 -- Rotational Damper/LConn1 -- Inertia12/LConn1 -- Input Shaft Even/RConn1 -- Gear2/LConn1 -- Gear6/LConn1
  PS-Simulink Converter1/LConn1 -- Synchronizer 3-1/RConn1
  Synchronizer 5-N/RConn1 -- PS-Simulink Converter2/LConn1
  PS-Simulink Converter/LConn1 -- Synchronizer 2-4/RConn1
  PS-Simulink Converter3/LConn1 -- Synchronizer R-6/RConn1
  Ideal Force Source/LConn1 -- Mass/LConn1 -- Synchronizer 2-4/LConn1
  Simulink-PS Converter1/RConn1 -- Ideal Force Source/RConn1
  Mechanical Translational Reference/LConn1 -- Ideal Force Source/RConn2
  Simulink-PS Converter2/RConn1 -- Ideal Force Source1/RConn1
  Mechanical Translational Reference1/LConn1 -- Ideal Force Source1/RConn2
  Ideal Force Source1/LConn1 -- Mass1/LConn1 -- Synchronizer 3-1/LConn1
  Ideal Force Source2/LConn1 -- Mass2/LConn1 -- Synchronizer R-6/LConn1
  Simulink-PS Converter3/RConn1 -- Ideal Force Source2/RConn1
  Mechanical Translational Reference2/LConn1 -- Ideal Force Source2/RConn2
  Ideal Force Source3/LConn1 -- Synchronizer 5-N/LConn1 -- Mass3/LConn1
  Simulink-PS Converter4/RConn1 -- Ideal Force Source3/RConn1
  Mechanical Translational Reference3/LConn1 -- Ideal Force Source3/RConn2
  Rotational Free End/LConn1 -- Synchronizer 5-N/RConn3 -- Inertia4/LConn1
  Syn 1 Delta Spd/RConn2 -- PS-Simulink Converter4/LConn1
  Syn 3 Delta Spd/RConn2 -- PS-Simulink Converter6/LConn1
  Syn 2 Delta Spd/RConn2 -- PS-Simulink Converter5/LConn1
  Syn 4 Delta Spd/RConn2 -- PS-Simulink Converter7/LConn1
  Syn 6 Delta Spd/RConn2 -- PS-Simulink Converter9/LConn1
  Syn R Delta Spd/RConn2 -- PS-Simulink Converter8/LConn1
  Syn 5 Delta Spd/RConn2 -- PS-Simulink Converter10/LConn1
  Mechanical Rotational Reference/LConn1 -- Rotational Damper/RConn1
  Mechanical Rotational Reference1/LConn1 -- Rotational Damper1/RConn1
  Mechanical Rotational Reference2/LConn1 -- Rotational Damper2/RConn1
  Mechanical Rotational Reference3/LConn1 -- Rotational Damper3/RConn1
  Mechanical Rotational Reference4/LConn1 -- Rotational Damper4/RConn1
  Ideal Rotational Motion Sensor2/RConn1 -- Mechanical Rotational Reference5/LConn1
  Ideal Rotational Motion Sensor2/RConn2 -- PS-Simulink Converter11/LConn1

== system MIL_VehicleTestEnvironment_MG_DCT_1/Shift Control System/Solenoid control ==
  target current : Inport
  Constant : Constant  Value=13/VBS1R*1000
  MinMax : MinMax  Inputs=2
  actual current : Outport  VectorParamsAs1DForOutWhenUnconnected=off
  wires:
  Constant/1 -> MinMax/2
  target current/1 -> MinMax/1
  MinMax/1 -> actual current/1

== system MIL_VehicleTestEnvironment_MG_DCT_1/Shift Control System/Solenoid control1 ==
  target current : Inport
  Constant : Constant  Value=13/VBS2R*1000
  MinMax : MinMax  Inputs=2
  actual current : Outport  VectorParamsAs1DForOutWhenUnconnected=off
  wires:
  Constant/1 -> MinMax/2
  target current/1 -> MinMax/1
  MinMax/1 -> actual current/1

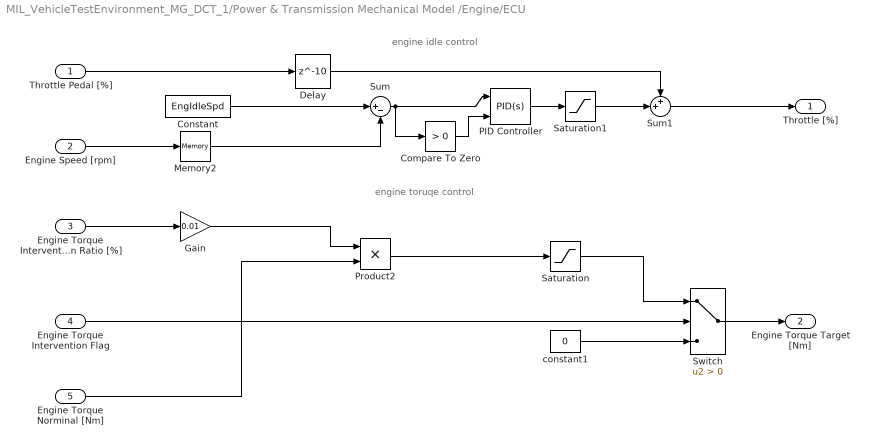
== system MIL_VehicleTestEnvironment_MG_DCT_1/Power & Transmission Mechanical Model /Engine/ECU ==
  note: engine idle control
  note: engine toruqe control
  Throttle Pedal [%] : Inport
  Engine Speed [rpm] : Inport  Port=2
  Engine Torque Intervention Ratio [%] : Inport  Port=3
  Engine Torque Intervention Flag : Inport  Port=4
  Engine Torque Norminal [Nm] : Inport  Port=5
  Compare To Zero : simulink/Logic and Bit Operations/Compare To Zero  relop=>  OutDataTypeStr=boolean
  Constant : Constant  Value=EngIdleSpd
  Delay : Delay  DelayLength=10
  Gain : Gain  Gain=0.01
  Memory2 : Memory  InitialCondition=EngIdleSpd
  PID Controller : simulink/Continuous/PID Controller  Controller=PID  Form=Parallel  TimeDomain=Continuous-time  SampleTime=-1  IntegratorMethod=Forward Euler  FilterMethod=Forward Euler  ControllerParametersSource=internal  P=0.1  I=0.5  D=0  UseFilter=on  N=100  TunerSelectOption=Transfer Function Based (PID Tuner App)  InitialConditionSource=internal  InitialConditionForIntegrator=0  InitialConditionForFilter=0  DifferentiatorICPrevScaledInput=0  ExternalReset=rising  TrackingMode=off  Kt=1  LimitOutput=off  UpperSaturationLimit=30  LowerSaturationLimit=0  LinearizeAsGain=off  AntiWindupMode=none  Kb=1  POutMin=[]  POutMax=[]  IOutMin=[]  IOutMax=[]  DOutMin=[]  DOutMax=[]  NOutMin=[]  NOutMax=[]  SumOutMin=[]  SumOutMax=[]  SaturationOutMin=[]  SaturationOutMax=[]  PParamMin=[]  PParamMax=[]  IParamMin=[]  IParamMax=[]  DParamMin=[]  DParamMax=[]  NParamMin=[]  NParamMax=[]  KbParamMin=[]  KbParamMax=[]  KtParamMin=[]  KtParamMax=[]  KbOutMin=[]  KbOutMax=[]  KtOutMin=[]  KtOutMax=[]  IntegratorOutMin=[]  IntegratorOutMax=[]  FilterOutMin=[]  FilterOutMax=[]  SumI1OutMin=[]  SumI1OutMax=[]  SumI2OutMin=[]  SumI2OutMax=[]  SumI3OutMin=[]  SumI3OutMax=[]  SumI4OutMin=[]  SumI4OutMax=[]  SumDOutMin=[]  SumDOutMax=[]  DifferentiatorOutMin=[]  DifferentiatorOutMax=[]  FilterDiffOutCoefMin=[]  FilterDiffOutCoefMax=[]  ReciprocalOutMin=[]  ReciprocalOutMax=[]  SumDenOutMin=[]  SumDenOutMax=[]  SumNumOutMin=[]  SumNumOutMax=[]  DivideOutMin=[]  DivideOutMax=[]  IntegratorContinuousStateAttributes=''  IntegratorStateMustResolveToSignalObject=off  IntegratorRTWStateStorageClass=Auto  FilterContinuousStateAttributes=''  FilterStateMustResolveToSignalObject=off  FilterRTWStateStorageClass=Auto  ParallelPVariant=InternalParameters  IdealPVariant=Disabled  IVariant=InternalParameters  DVariant=InternalParameters  IntegratorVariant=Continuous  SatVariant=Disabled  AWVariant=Passthrough  PCopyVariant=Disabled  TRVariant=Disabled  FdbkBlocksVariant=Forward  IdealPFdbkVariant=Disabled  SatFdbkVariant=Disabled  DerivativeFilterVariant=ContFilter  NVariant=InternalParameters  NCopyVariant=Disabled  FilterICVariant=InternalICsFilter  IntegratorICVariant=InternalICs  ExternalResetVariant=ExternalReset  TRSumVariant=Passthrough  SumFdbkVariant=Disabled  SumVariant=Sum_PID
  Product2 : Product  RndMeth=Zero
  Saturation : Saturate  UpperLimit=EngTqMax  LowerLimit=0
  Saturation1 : Saturate  UpperLimit=0  LowerLimit=0
  Sum : Sum  Inputs=|+-
  Sum1 : Sum  Inputs=++|
  Switch : Switch  Criteria=u2 > Threshold
  constant1 : Constant  Value=0
  Throttle [%] : Outport  VectorParamsAs1DForOutWhenUnconnected=off
  "Engine Torque Target [Nm] " : Outport  Port=2  VectorParamsAs1DForOutWhenUnconnected=off
  wires:
  Engine Speed [rpm]/1 -> Memory2/1
  Constant/1 -> Sum/1
  Sum/1 -> Compare To Zero/1, PID Controller/1
  Gain/1 -> Product2/1
  Engine Torque Norminal [Nm]/1 -> Product2/2
  Saturation/1 -> Switch/1
  Engine Torque Intervention Ratio [%]/1 -> Gain/1
  Product2/1 -> Saturation/1
  Engine Torque Intervention Flag/1 -> Switch/2
  Throttle Pedal [%]/1 -> Delay/1
  Sum1/1 -> Throttle [%]/1
  constant1/1 -> Switch/3
  Switch/1 -> "Engine Torque Target [Nm] "/1
  Memory2/1 -> Sum/2
  PID Controller/1 -> Saturation1/1
  Saturation1/1 -> Sum1/2
  Compare To Zero/1 -> PID Controller/2
  Delay/1 -> Sum1/1

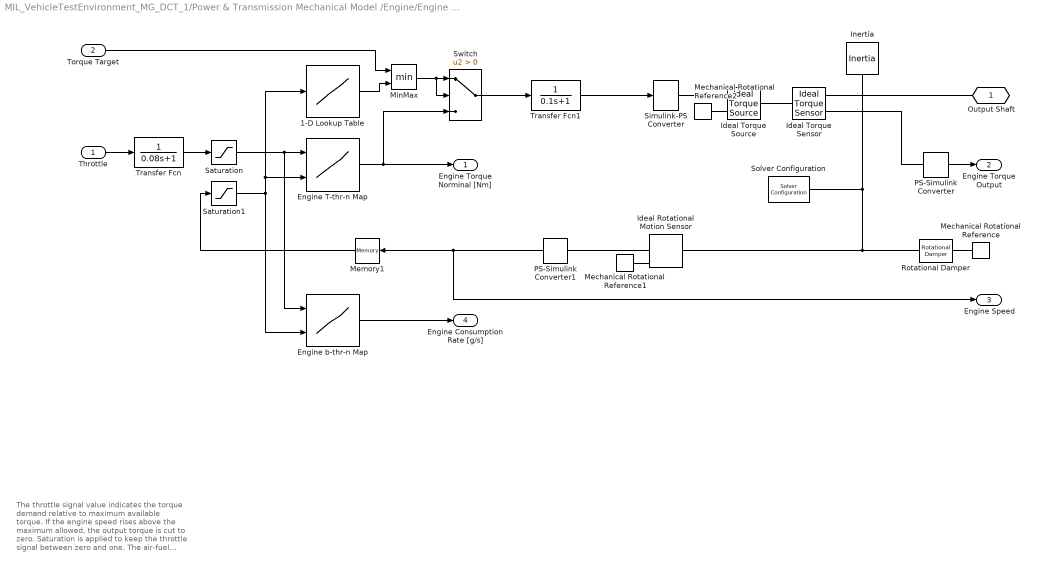
== system MIL_VehicleTestEnvironment_MG_DCT_1/Power & Transmission Mechanical Model /Engine/Engine Main ==
  note: The throttle signal value indicates the torque demand
      | relative to maximum available torque. If the engine
      | speed rises above the maximum allowed, the output
      | torque is cut to zero. Saturation is applied to keep the
      | throttle signal between zero and one.
      |
      | The air-fuel combustion dynamics is not modeled.
  Throttle : Inport
  Torque Target : Inport  Port=2
  1-D Lookup Table : Lookup_n-D  NumberOfTableDimensions=1  BreakpointsForDimension1=EngTqMapSpdIndx  Table=EngTqExtChartc  ExtrapMethod=Clip  UseLastTableValue=on  InternalRulePriority=Speed  RndMeth=Simplest  InputSameDT=on
  Engine T-thr-n Map : Lookup_n-D  BreakpointsForDimension1=EngTqMapThrtIndx  BreakpointsForDimension2=EngTqMapSpdIndx  Table=EngTqMapTq  ExtrapMethod=Clip  UseLastTableValue=on  RndMeth=Simplest  InputSameDT=on
  Engine b-thr-n Map : Lookup_n-D  BreakpointsForDimension1=EngFuelCnsPerSecMapThrtIndx  BreakpointsForDimension2=EngFuelCnsPerSecMapSpdIndx  Table=EngFuelCnsPerSecMapCns  ExtrapMethod=Clip  UseLastTableValue=on  RndMeth=Simplest  InputSameDT=on
  Ideal Rotational Motion Sensor : fl_lib/Mechanical/Mechanical Sensors/Ideal Rotational Motion Sensor  wrap_angle=simscape.enum.onoff.off  offset=0 rad
  Ideal Torque Sensor : fl_lib/Mechanical/Mechanical Sensors/Ideal Torque Sensor
  Ideal Torque Source : fl_lib/Mechanical/Mechanical Sources/Ideal Torque Source
  Inertia : fl_lib/Mechanical/Rotational Elements/Inertia  inertia=EngInrt kg*m^2  w_specify=on  w_priority=High  w=EngIdleSpd*2 rpm  w_nominal_specify=off  w_nominal_unit=rad/s  w_nominal_value=1  t_specify=off  t_priority=High  t=0 N*m  t_nominal_specify=off  t_nominal_unit=N*m  t_nominal_value=1
  Mechanical Rotational Reference : fl_lib/Mechanical/Rotational Elements/Mechanical Rotational Reference
  Mechanical Rotational Reference1 : fl_lib/Mechanical/Rotational Elements/Mechanical Rotational Reference
  Mechanical Rotational Reference2 : fl_lib/Mechanical/Rotational Elements/Mechanical Rotational Reference
  Memory1 : Memory
  MinMax : MinMax  Inputs=2
  PS-Simulink Converter : nesl_utility/PS-Simulink Converter  PhysicalDomain=network_engine_domain  SubClassName=ps_output  LeftPortType=input  RightPortType=output  PseudoPeriodic=off  Frequencies=[]  Unit=N*m  AffineConversion=off
  PS-Simulink Converter1 : nesl_utility/PS-Simulink Converter  PhysicalDomain=network_engine_domain  SubClassName=ps_output  LeftPortType=input  RightPortType=output  PseudoPeriodic=off  Frequencies=[]  Unit=rpm  AffineConversion=off
  Rotational Damper : fl_lib/Mechanical/Rotational Elements/Rotational Damper  D=0 N*m/(rad/s)  w_specify=off  w_priority=High  w=0 rad/s  w_nominal_specify=off  w_nominal_unit=rad/s  w_nominal_value=1  t_specify=off  t_priority=High  t=0 N*m  t_nominal_specify=off  t_nominal_unit=N*m  t_nominal_value=1
  Saturation : Saturate  UpperLimit=100  LowerLimit=0.0
  Saturation1 : Saturate  UpperLimit=EngSpdMax  LowerLimit=0
  Simulink-PS Converter : nesl_utility/Simulink-PS Converter  PhysicalDomain=network_engine_domain  SubClassName=ps_input  LeftPortType=input  RightPortType=output  PseudoPeriodic=off  Frequencies=[]  NoiseDistribution=none  NoiseParameters=[]  Unit=N*m  AffineConversion=off  FilteringAndDerivatives=zero  SimscapeFilterOrder=1  InputFilterTimeConstant=0.001  UdotUserProvided=1
  Solver Configuration : nesl_utility/Solver Configuration  PhysicalDomain=network_engine_domain  SubClassName=solver  LeftPortType=input  RightPortType=generic  Tones=[]  Harmonics=[]  SimulateNoise=off  Profile=off  UseLocalSampling=off  EnableSwitchedLinearOptims=on  FrequencyDomain=off  UseCCode=off  RelTol=0.001  AbsTol=1e-06  MinStep=1e-09  ToWorkspace=off  RevertToSquareIcSolve=off  NumHomotopyIterations=100  PhasorMode=off  PhasorModeNumHarmonics=1  DoDC=off  ResidualTolerance=1e-09  UseLocalSolver=on  LocalSolverChoice=NE_TRAPEZOIDAL_ADVANCER  LocalSolverSampleTime=0.001  DoFixedCost=on  MaxNonlinIter=3  MaxModeIter=2  LinearAlgebra=Sparse  EquationFormulation=NE_TIME_EF  DelaysMemoryBudget=1024  AutomaticFiltering=on  FilteringTimeConstant=0.001  PartitionStorageMethod=AS_NEEDED  PartitionMemoryBudget=1024  PartitionMethod=FAST
  Switch : Switch  Criteria=u2 > Threshold
  Transfer Fcn : TransferFcn  Denominator=[0.08 1]
  Transfer Fcn1 : TransferFcn  Denominator=[0.1 1]
  Output Shaft : PMIOPort  Side=Right
  Engine Torque Norminal [Nm] : Outport  VectorParamsAs1DForOutWhenUnconnected=off
  Engine Torque Output : Outport  Port=2  VectorParamsAs1DForOutWhenUnconnected=off
  Engine Speed : Outport  Port=3  VectorParamsAs1DForOutWhenUnconnected=off
  Engine Consumption Rate [g/s] : Outport  Port=4  VectorParamsAs1DForOutWhenUnconnected=off
  wires:
  PS-Simulink Converter1/1 -> Engine Speed/1, Memory1/1
  Throttle/1 -> Transfer Fcn/1
  Switch/1 -> Transfer Fcn1/1
  Engine T-thr-n Map/1 -> Switch/3, Engine Torque Norminal [Nm]/1
  Memory1/1 -> Saturation1/1
  Saturation1/1 -> Engine b-thr-n Map/2, 1-D Lookup Table/1, Engine T-thr-n Map/2
  1-D Lookup Table/1 -> MinMax/2
  MinMax/1 -> Switch/2, Switch/1
  Transfer Fcn1/1 -> Simulink-PS Converter/1
  Torque Target/1 -> MinMax/1
  Transfer Fcn/1 -> Saturation/1
  Saturation/1 -> Engine b-thr-n Map/1, Engine T-thr-n Map/1
  Engine b-thr-n Map/1 -> Engine Consumption Rate [g/s]/1
  PS-Simulink Converter/1 -> Engine Torque Output/1
  connections:
  Ideal Torque Source/RConn1 -- Simulink-PS Converter/RConn1
  PS-Simulink Converter/LConn1 -- Ideal Torque Sensor/RConn2
  Rotational Damper/LConn1 -- Ideal Rotational Motion Sensor/LConn1 -- Output Shaft/RConn1 -- Ideal Torque Sensor/RConn1 -- Inertia/LConn1 -- Solver Configuration/RConn1
  PS-Simulink Converter1/LConn1 -- Ideal Rotational Motion Sensor/RConn2
  Mechanical Rotational Reference1/LConn1 -- Ideal Rotational Motion Sensor/RConn1
  Mechanical Rotational Reference2/LConn1 -- Ideal Torque Source/RConn2
  Mechanical Rotational Reference/LConn1 -- Rotational Damper/RConn1
  Ideal Torque Sensor/LConn1 -- Ideal Torque Source/LConn1

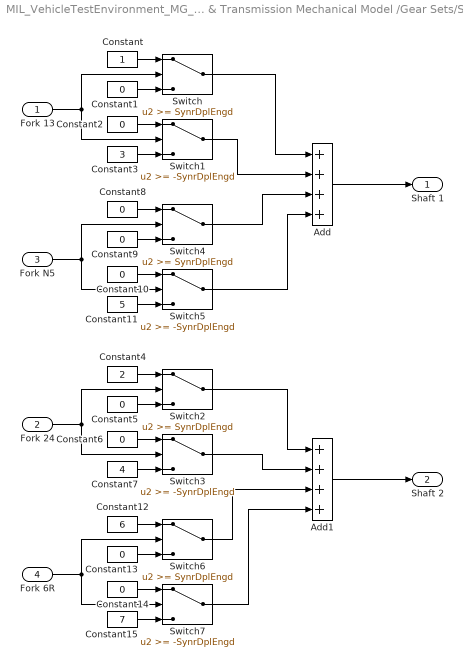
== system MIL_VehicleTestEnvironment_MG_DCT_1/Power & Transmission Mechanical Model /Gear Sets/Shaft Gear Judge  ==
  Fork 13 : Inport
  Fork 24 : Inport  Port=2
  Fork N5 : Inport  Port=3
  Fork 6R : Inport  Port=4
  Add : Sum  Inputs=++++
  Add1 : Sum  Inputs=++++
  Constant : Constant
  Constant{1..2,5..6,8..10,13..14} (9 alike) : Constant  Value=0
  Constant11 : Constant  Value=5
  Constant12 : Constant  Value=6
  Constant15 : Constant  Value=7
  Constant3 : Constant  Value=3
  Constant4 : Constant  Value=2
  Constant7 : Constant  Value=4
  Switch{,2,4,6} (4 alike) : Switch  Threshold=SynrDplEngd
  Switch{1,3,5,7} (4 alike) : Switch  Threshold=-SynrDplEngd
  Shaft 1 : Outport  VectorParamsAs1DForOutWhenUnconnected=off
  Shaft 2 : Outport  Port=2  VectorParamsAs1DForOutWhenUnconnected=off
  wires:
  Constant1/1 -> Switch/3
  Constant/1 -> Switch/1
  Add/1 -> Shaft 1/1
  Fork 13/1 -> Switch/2, Switch1/2
  Switch3/1 -> Add1/2
  Add1/1 -> Shaft 2/1
  Switch5/1 -> Add/4
  Switch4/1 -> Add/3
  Fork 6R/1 -> Switch7/2, Switch6/2
  Switch/1 -> Add/1
  Constant10/1 -> Switch5/1
  Constant4/1 -> Switch2/1
  Switch1/1 -> Add/2
  Switch6/1 -> Add1/3
  Constant11/1 -> Switch5/3
  Fork N5/1 -> Switch4/2, Switch5/2
  Constant12/1 -> Switch6/1
  Constant6/1 -> Switch3/1
  Fork 24/1 -> Switch3/2, Switch2/2
  Constant9/1 -> Switch4/3
  Switch7/1 -> Add1/4
  Constant3/1 -> Switch1/3
  Switch2/1 -> Add1/1
  Constant8/1 -> Switch4/1
  Constant14/1 -> Switch7/1
  Constant2/1 -> Switch1/1
  Constant13/1 -> Switch6/3
  Constant5/1 -> Switch2/3
  Constant7/1 -> Switch3/3
  Constant15/1 -> Switch7/3

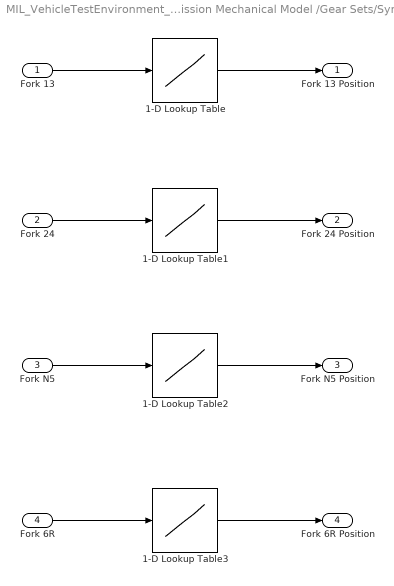
== system MIL_VehicleTestEnvironment_MG_DCT_1/Power & Transmission Mechanical Model /Gear Sets/Synchronizer position signal transfer ==
  Fork 13 : Inport
  Fork 24 : Inport  Port=2
  Fork N5 : Inport  Port=3
  Fork 6R : Inport  Port=4
  1-D Lookup Table : Lookup_n-D  NumberOfTableDimensions=1  BreakpointsForDimension1=[-SynrDplFinshd,-SynrDplSync,0,SynrDplSync,SynrDplFinshd]  Table=[Fork1PosnB,Fork1PosnSyncB,Fork1PosnNeut,Fork1PosnSyncA,Fork1PosnA]  InternalRulePriority=Speed  RndMeth=Simplest  InputSameDT=on
  1-D Lookup Table1 : Lookup_n-D  NumberOfTableDimensions=1  BreakpointsForDimension1=[-SynrDplFinshd,-SynrDplSync,0,SynrDplSync,SynrDplFinshd]  Table=[Fork2PosnB,Fork2PosnSyncB,Fork2PosnNeut,Fork2PosnSyncA,Fork2PosnA]  InternalRulePriority=Speed  RndMeth=Simplest  InputSameDT=on
  1-D Lookup Table2 : Lookup_n-D  NumberOfTableDimensions=1  BreakpointsForDimension1=[-SynrDplFinshd,-SynrDplSync,0,SynrDplSync,SynrDplFinshd]  Table=[Fork3PosnB,Fork3PosnSyncB,Fork3PosnNeut,Fork3PosnSyncA,Fork3PosnA]  InternalRulePriority=Speed  RndMeth=Simplest  InputSameDT=on
  1-D Lookup Table3 : Lookup_n-D  NumberOfTableDimensions=1  BreakpointsForDimension1=[-SynrDplFinshd,-SynrDplSync,0,SynrDplSync,SynrDplFinshd]  Table=[Fork4PosnB,Fork4PosnSyncB,Fork4PosnNeut,Fork4PosnSyncA,Fork4PosnA]  InternalRulePriority=Speed  RndMeth=Simplest  InputSameDT=on
  Fork 13 Position : Outport  VectorParamsAs1DForOutWhenUnconnected=off
  Fork 24 Position : Outport  Port=2  VectorParamsAs1DForOutWhenUnconnected=off
  Fork N5 Position : Outport  Port=3  VectorParamsAs1DForOutWhenUnconnected=off
  Fork 6R Position : Outport  Port=4  VectorParamsAs1DForOutWhenUnconnected=off
  wires:
  1-D Lookup Table/1 -> Fork 13 Position/1
  1-D Lookup Table1/1 -> Fork 24 Position/1
  1-D Lookup Table2/1 -> Fork N5 Position/1
  1-D Lookup Table3/1 -> Fork 6R Position/1
  Fork 13/1 -> 1-D Lookup Table/1
  Fork 24/1 -> 1-D Lookup Table1/1
  Fork N5/1 -> 1-D Lookup Table2/1
  Fork 6R/1 -> 1-D Lookup Table3/1
